simulink model "mod"  (R2014b)
settings: Solver=ode4  StartTime=0.0  StopTime=100  FixedStep=tp  MaxStep=2  MinStep=0.01  RelTol=1e-3
values from neighbouring files (symbols this model uses):
  k = 8    [Untitled.m]
  tp = 10    [Untitled.m]
settings Model: Creator=podstawy  LastModifiedBy=podstawy

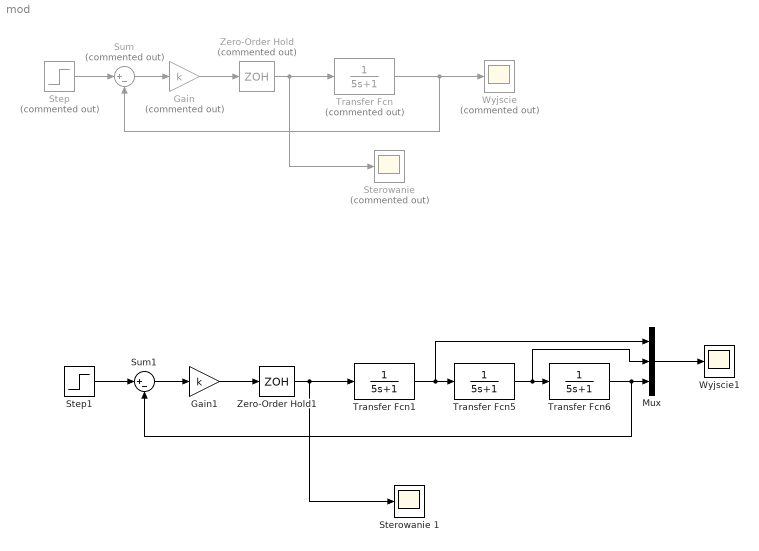
== system mod ==
  Gain : Gain  Commented=on  Gain=k
  Gain1 : Gain  Gain=k
  Mux : Mux  Inputs=3
  Step : Step  Commented=on  SampleTime=0
  Step1 : Step  SampleTime=0
  "Sterowanie " : Scope  Commented=on
      settings: SaveName=s
  Sterowanie 1 : Scope
      settings: SaveName=s1
  Sum : Sum  Commented=on  Inputs=|+-
  Sum1 : Sum  Inputs=|+-
  Transfer Fcn : TransferFcn  Commented=on  Denominator=[5 1]
  Transfer Fcn1 : TransferFcn  Denominator=[5 1]
  Transfer Fcn5 : TransferFcn  Denominator=[5 1]
  Transfer Fcn6 : TransferFcn  Denominator=[5 1]
  Wyjscie : Scope  Commented=on
      settings: SaveName=w
  Wyjscie1 : Scope
      settings: SaveName=w1
  Zero-Order Hold : ZeroOrderHold  Commented=on  SampleTime=tp
  Zero-Order Hold1 : ZeroOrderHold  SampleTime=tp
  wires:
  Gain/1 -> Zero-Order Hold/1
  Zero-Order Hold/1 -> "Sterowanie "/1, Transfer Fcn/1
  Sum/1 -> Gain/1
  Transfer Fcn/1 -> Sum/2, Wyjscie/1
  Step/1 -> Sum/1
  Gain1/1 -> Zero-Order Hold1/1
  Zero-Order Hold1/1 -> Sterowanie 1/1, Transfer Fcn1/1
  Sum1/1 -> Gain1/1
  Step1/1 -> Sum1/1
  Transfer Fcn5/1 -> Mux/2, Transfer Fcn6/1
  Transfer Fcn1/1 -> Mux/1, Transfer Fcn5/1
  Transfer Fcn6/1 -> Sum1/2, Mux/3
  Mux/1 -> Wyjscie1/1
